simulink model "IEEE33_SmartInverter_Physical"  (R2026a)
settings: Solver=ode23t  StopTime=2.4  MaxStep=1e-3
PreLoadFcn:
  | try, startup_project(); addpath(fullfile(pwd,'simulink_physical')); if evalin('base','exist(''simscape_pv_p_commands'',''var'')') == 0, prepare_ieee33_simscape_inputs(80,'partial_cloud','hybrid'); end; catch ME, disp(['Physical-model preload warning: ' ME.message]); end
undefined symbols (not defined in the file or in its folder): simscape_pv_capacity_kW
libraries: ee_lib x116, nesl_utility x111, fl_lib x34
(part 1 of 2)
settings Model: Creator=ismahin  LastModifiedBy=ismahin

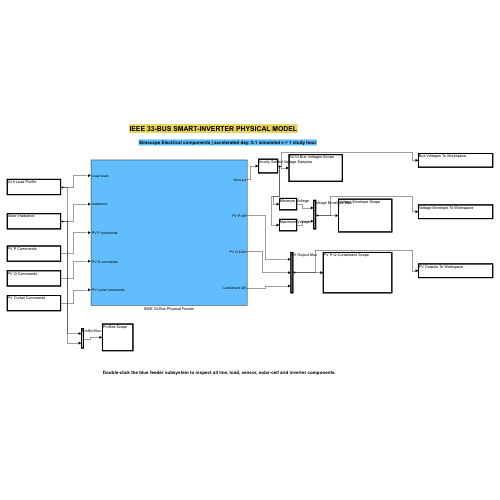
[thumbnail: Simulink's stored preview of the top-level diagram]
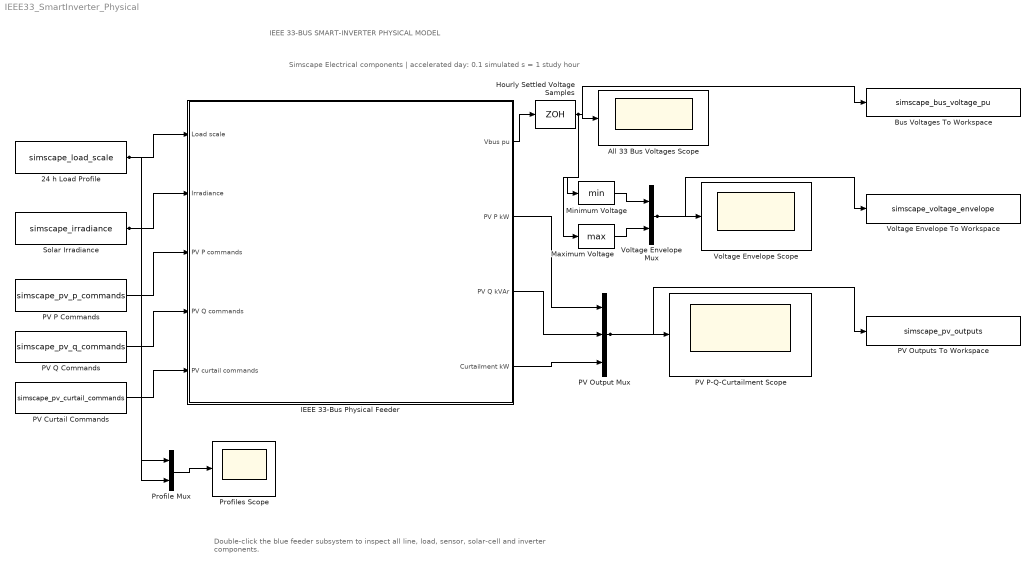
== system IEEE33_SmartInverter_Physical ==
  note: IEEE 33-BUS SMART-INVERTER PHYSICAL MODEL
  note: Simscape Electrical components | accelerated day: 0.1 simulated s = 1 study hour
  note: Double-click the blue feeder subsystem to inspect all line, load, sensor, solar-cell and inverter components.
  24 h Load Profile : FromWorkspace  VariableName=simscape_load_scale  OutputAfterFinalValue=Holding final value
  All 33 Bus Voltages Scope : Scope
      settings: TimeSpan=2.4  ActiveDisplayYMinimum=0.85  ActiveDisplayYMaximum=1.15  YLabel=Voltage (p.u.)
  Bus Voltages To Workspace : ToWorkspace  VariableName=simscape_bus_voltage_pu  SaveFormat=Timeseries  SampleTime=-1
      settings: MaxDataPoints=20000
  Hourly Settled Voltage Samples : ZeroOrderHold  SampleTime=[0.1 0.085]
  IEEE 33-Bus Physical Feeder : Subsystem
  Maximum Voltage : MinMax  Function=max
  Minimum Voltage : MinMax
  PV Curtail Commands : FromWorkspace  VariableName=simscape_pv_curtail_commands  OutputAfterFinalValue=Holding final value
  PV Output Mux : Mux  Inputs=3
  PV Outputs To Workspace : ToWorkspace  VariableName=simscape_pv_outputs  SaveFormat=Timeseries  SampleTime=-1
      settings: MaxDataPoints=20000
  PV P Commands : FromWorkspace  VariableName=simscape_pv_p_commands  OutputAfterFinalValue=Holding final value
  PV P-Q-Curtailment Scope : Scope
      settings: TimeSpan=2.4  YLabel=kW / kVAr
  PV Q Commands : FromWorkspace  VariableName=simscape_pv_q_commands  OutputAfterFinalValue=Holding final value
  Profile Mux : Mux  Inputs=2
  Profiles Scope : Scope
      settings: TimeSpan=2.4  YLabel=Load / irradiance (p.u.)
  Solar Irradiance : FromWorkspace  VariableName=simscape_irradiance  OutputAfterFinalValue=Holding final value
  Voltage Envelope Mux : Mux  Inputs=2
  Voltage Envelope Scope : Scope
      settings: TimeSpan=2.4  ActiveDisplayYMinimum=0.85  ActiveDisplayYMaximum=1.15  YLabel=Min / max voltage (p.u.)
  Voltage Envelope To Workspace : ToWorkspace  VariableName=simscape_voltage_envelope  SaveFormat=Timeseries  SampleTime=-1
      settings: MaxDataPoints=20000
  wires:
  24 h Load Profile/1 -> IEEE 33-Bus Physical Feeder/1(Load scale), Profile Mux/1
  Solar Irradiance/1 -> IEEE 33-Bus Physical Feeder/2(Irradiance), Profile Mux/2
  PV P Commands/1 -> IEEE 33-Bus Physical Feeder/3(PV P commands)
  PV Q Commands/1 -> IEEE 33-Bus Physical Feeder/4(PV Q commands)
  PV Curtail Commands/1 -> IEEE 33-Bus Physical Feeder/5(PV curtail commands)
  Profile Mux/1 -> Profiles Scope/1
  IEEE 33-Bus Physical Feeder/1(Vbus pu) -> Hourly Settled Voltage Samples/1
  Hourly Settled Voltage Samples/1 -> All 33 Bus Voltages Scope/1, Minimum Voltage/1, Maximum Voltage/1, Bus Voltages To Workspace/1
  Minimum Voltage/1 -> Voltage Envelope Mux/1
  Maximum Voltage/1 -> Voltage Envelope Mux/2
  Voltage Envelope Mux/1 -> Voltage Envelope Scope/1, Voltage Envelope To Workspace/1
  IEEE 33-Bus Physical Feeder/2(PV P kW) -> PV Output Mux/1
  IEEE 33-Bus Physical Feeder/3(PV Q kVAr) -> PV Output Mux/2
  IEEE 33-Bus Physical Feeder/4(Curtailment kW) -> PV Output Mux/3
  PV Output Mux/1 -> PV P-Q-Curtailment Scope/1, PV Outputs To Workspace/1
